simulink model "Lead_Tustin_2a_ordem"  (R2019b)
settings: Solver=VariableStepAuto  StartTime=0.0  StopTime=3  RelTol=1e-3
settings Model: Creator=fernandopassold  LastModifiedBy=fernandopassold

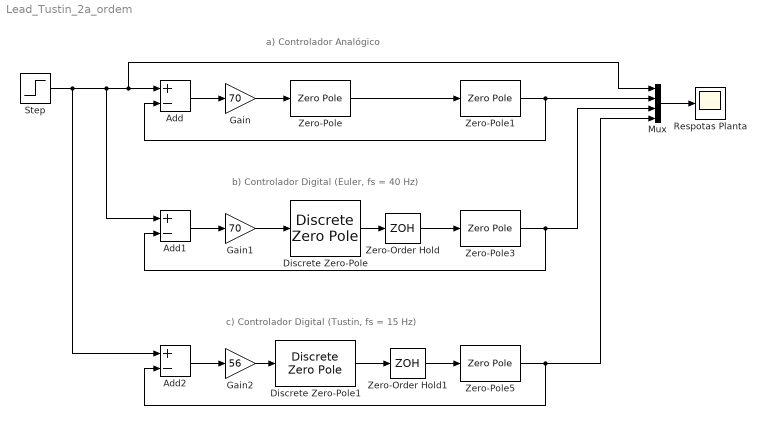
== system Lead_Tustin_2a_ordem ==
  note: a) Controlador Analógico
  note: b) Controlador Digital (Euler, fs = 40 Hz)
  note: c) Controlador Digital (Tustin, fs = 15 Hz)
  Add : Sum  Inputs=+-
  Add1 : Sum  Inputs=+-
  Add2 : Sum  Inputs=+-
  Discrete Zero-Pole : DiscreteZeroPole  Zeros=[ 0.95]  Poles=[0.75]  Gain=1  SampleTime=1/40
  Discrete Zero-Pole1 : DiscreteZeroPole  Zeros=[0.875]  Poles=[0.5]  Gain=1  SampleTime=1/15
  Gain : Gain  Gain=70
  Gain1 : Gain  Gain=70
  Gain2 : Gain  Gain=56
  Mux : Mux
  Respotas Planta : Scope
  Step : Step  SampleTime=0
  Zero-Order Hold : ZeroOrderHold  SampleTime=1/40
  Zero-Order Hold1 : ZeroOrderHold  SampleTime=1/15
  Zero-Pole : ZeroPole  Zeros=[-2]  Poles=[-10]
  Zero-Pole1 : ZeroPole  Zeros=[ ]  Poles=[0 -1]
  Zero-Pole3 : ZeroPole  Zeros=[ ]  Poles=[0 -1]
  Zero-Pole5 : ZeroPole  Zeros=[ ]  Poles=[0 -1]
  wires:
  Add/1 -> Gain/1
  Gain/1 -> Zero-Pole/1
  Zero-Pole/1 -> Zero-Pole1/1
  Zero-Pole1/1 -> Add/2, Mux/2
  Step/1 -> Add2/1, Add1/1, Mux/1, Add/1
  Add1/1 -> Gain1/1
  Gain1/1 -> Discrete Zero-Pole/1
  Zero-Pole3/1 -> Add1/2, Mux/3
  Add2/1 -> Gain2/1
  Gain2/1 -> Discrete Zero-Pole1/1
  Zero-Pole5/1 -> Add2/2, Mux/4
  Discrete Zero-Pole/1 -> Zero-Order Hold/1
  Zero-Order Hold/1 -> Zero-Pole3/1
  Discrete Zero-Pole1/1 -> Zero-Order Hold1/1
  Zero-Order Hold1/1 -> Zero-Pole5/1
  Mux/1 -> Respotas Planta/1
